simulink subsystem "TrajectoryLinkController"  (R2022b)
settings: Solver=VariableStepAuto  StartTime=0.0  StopTime=10.0  RelTol=1e-3
model mask{Tsampling=Tsampling, KpDiscrete=K(1,1), KdDiscrete=K(1,2), KiDiscrete=K(1,3), KpContinuous=K(1,1), KdContinuous=K(1,2), KiContinuous=K(1,3), ContinuousController=on}
  mask prompts: ContinuousController "Simulate Continuous Controller"
values from neighbouring files (symbols this model uses):
  Tsampling = 1e-3    (= 0.001)    [SimulationInput.m]    (also in SimulinkParameters.m; overleaf_sim.m; test_my_sim_class.m)
libraries: slpidlib x1
settings Model: Creator=papaveneti  LastModifiedBy=papaveneti

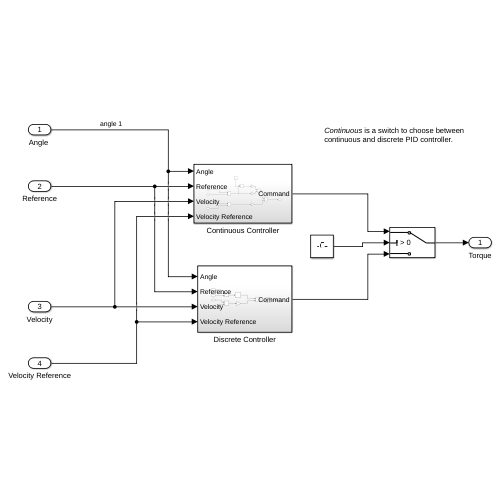
[thumbnail: Simulink's stored preview of the top-level diagram]
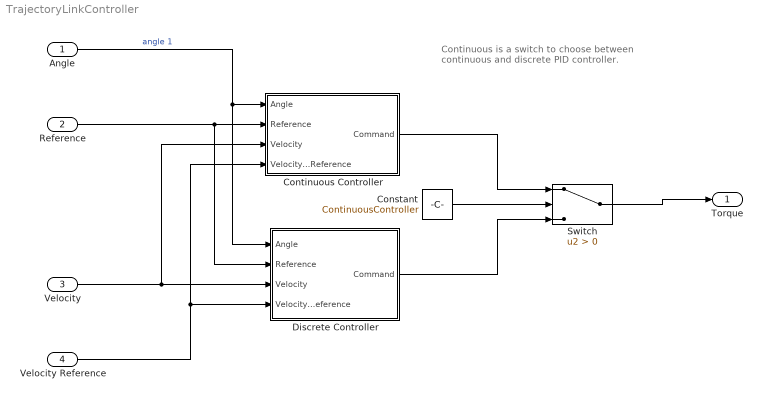
== system TrajectoryLinkController ==
  note: Continuous is a switch to choose between
      | continuous and discrete PID controller.
  "Angle " : Inport
  Reference : Inport  Port=2
  Velocity : Inport  Port=3
  Velocity Reference : Inport  Port=4
  Constant : Constant  Value=ContinuousController
  Continuous Controller : Subsystem
  Discrete Controller : Subsystem
  Switch : Switch  Criteria=u2 > Threshold  SaturateOnIntegerOverflow=off  InputSameDT=off
  Torque : Outport
  wires:
  Velocity Reference/1 -> Continuous Controller/4(Velocity Reference), Discrete Controller/4(Velocity Reference)
  Reference/1 -> Continuous Controller/2(Reference), Discrete Controller/2(Reference)
  Discrete Controller/1(Command) -> Switch/3
  Switch/1 -> Torque/1
  Continuous Controller/1(Command) -> Switch/1
  Velocity/1 -> Discrete Controller/3(Velocity), Continuous Controller/3(Velocity)
  "Angle "/1 -> Continuous Controller/1("Angle "), Discrete Controller/1(Angle)  "angle 1"
  Constant/1 -> Switch/2

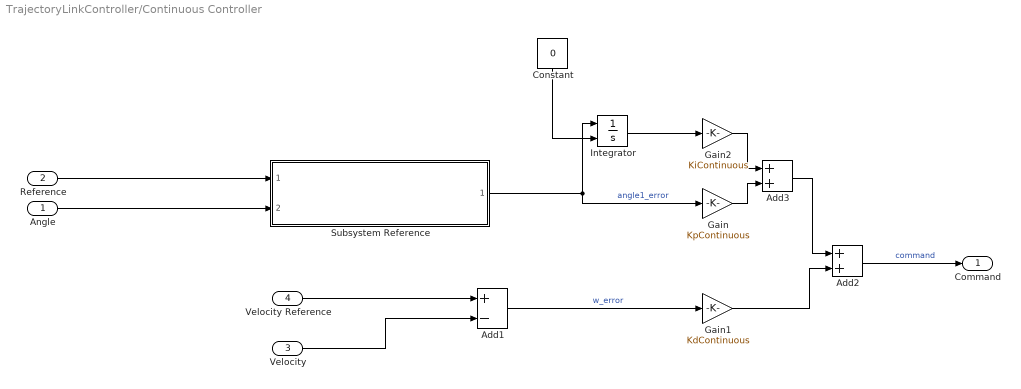
== system TrajectoryLinkController/Continuous Controller ==
  "Angle " : Inport
  Reference : Inport  Port=2
  Velocity : Inport  Port=3
  Velocity Reference : Inport  Port=4
  Add1 : Sum  Inputs=+-
  Add2 : Sum
  Add3 : Sum
  Constant : Constant  Value=0
  Gain : Gain  Gain=KpContinuous
  Gain1 : Gain  Gain=KdContinuous
  Gain2 : Gain  Gain=KiContinuous
  Integrator : Integrator  InitialConditionSource=external
  Subsystem Reference : Subsystem  ReferencedSubsystem=shortest_angle_diff
  Command : Outport
  wires:
  Constant/1 -> Integrator/2
  Add3/1 -> Add2/1
  Gain/1 -> Add3/2
  Gain2/1 -> Add3/1
  Integrator/1 -> Gain2/1
  Velocity Reference/1 -> Add1/1
  Velocity/1 -> Add1/2
  Subsystem Reference/1 -> Integrator/1, Gain/1  "angle1_error"
  "Angle "/1 -> Subsystem Reference/2
  Add2/1 -> Command/1  "command"
  Gain1/1 -> Add2/2
  Add1/1 -> Gain1/1  "w_error"
  Reference/1 -> Subsystem Reference/1

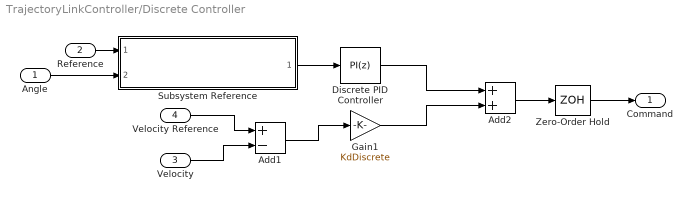
== system TrajectoryLinkController/Discrete Controller ==
  Angle : Inport
  Reference : Inport  Port=2
  Velocity : Inport  Port=3
  Velocity Reference : Inport  Port=4
  Add1 : Sum  Inputs=+-
  Add2 : Sum
  Discrete PID Controller : slpidlib/PID Controller  Controller=PI  Form=Parallel  TimeDomain=Discrete-time  UseExternalTs=off  SampleTime=Tsampling  IntegratorMethod=Forward Euler  FilterMethod=Forward Euler  ControllerParametersSource=internal  P=KpDiscrete  I=KiDiscrete  UseKiTs=off  D=0  N=100  UseFilter=off  TunerSelectOption=Transfer Function Based (PID Tuner App)  InitialConditionSource=internal  InitialConditionForIntegrator=0  InitialConditionForFilter=0  DifferentiatorICPrevScaledInput=0  ExternalReset=none  TrackingMode=off  Kt=1  LimitOutput=off  SatLimitsSource=internal  UpperSaturationLimit=inf  LowerSaturationLimit=-inf  LinearizeAsGain=off  AntiWindupMode=none  Kb=1  LimitIntegrator=off  UpperIntegratorSaturationLimit=inf  LowerIntegratorSaturationLimit=-inf  POutMin=[]  POutMax=[]  IOutMin=[]  IOutMax=[]  DOutMin=[]  DOutMax=[]  NOutMin=[]  NOutMax=[]  SumOutMin=[]  SumOutMax=[]  SaturationOutMin=[]  SaturationOutMax=[]  PParamMin=[]  PParamMax=[]  IParamMin=[]  IParamMax=[]  DParamMin=[]  DParamMax=[]  NParamMin=[]  NParamMax=[]  KbParamMin=[]  KbParamMax=[]  KtParamMin=[]  KtParamMax=[]  KbOutMin=[]  KbOutMax=[]  KtOutMin=[]  KtOutMax=[]  IntegratorOutMin=[]  IntegratorOutMax=[]  FilterOutMin=[]  FilterOutMax=[]  SumI1OutMin=[]  SumI1OutMax=[]  SumI2OutMin=[]  SumI2OutMax=[]  SumI3OutMin=[]  SumI3OutMax=[]  SumI4OutMin=[]  SumI4OutMax=[]  SumDOutMin=[]  SumDOutMax=[]  DifferentiatorOutMin=[]  DifferentiatorOutMax=[]  FilterDiffOutCoefMin=[]  FilterDiffOutCoefMax=[]  ReciprocalOutMin=[]  ReciprocalOutMax=[]  SumDenOutMin=[]  SumDenOutMax=[]  SumNumOutMin=[]  SumNumOutMax=[]  DivideOutMin=[]  DivideOutMax=[]  UdiffTsProdOutMin=[]  UdiffTsProdOutMax=[]  NTsProdOutMin=[]  NTsProdOutMax=[]  UintegralTsProdOutMin=[]  UintegralTsProdOutMax=[]  UngainTsProdOutMin=[]  UngainTsProdOutMax=[]  ClampingZeroOutDataTypeStr=Inherit: Inherit via back propagation  ClampingZeroOutMin=[]  ClampingZeroOutMax=[]  FilterDenConstantOutDataTypeStr=Inherit: Inherit via back propagation  FilterDenConstantOutMin=[]  FilterDenConstantOutMax=[]  PCopyOutDataTypeStr=Inherit: Inherit via back propagation  PCopyOutMin=[]  PCopyOutMax=[]  NCopyOutDataTypeStr=Inherit: Inherit via back propagation  NCopyOutMin=[]  NCopyOutMax=[]  IntegratorContinuousStateAttributes=''  IntegratorStateMustResolveToSignalObject=off  IntegratorRTWStateStorageClass=Auto  FilterContinuousStateAttributes=''  FilterStateMustResolveToSignalObject=off  FilterRTWStateStorageClass=Auto  ParallelPVariant=InternalParameters  IdealPVariant=Disabled  IVariant=InternalParameters  DVariant=Disabled  IntegratorVariant=Discrete  SatVariant=Disabled  AWVariant=Passthrough  PCopyVariant=Disabled  TRVariant=Disabled  FdbkBlocksVariant=Forward  IdealPFdbkVariant=Disabled  SatFdbkVariant=Disabled  DerivativeFilterVariant=Disabled  NVariant=Disabled  NCopyVariant=Disabled_SignalSpec  FilterICVariant=Disabled  IntegratorICVariant=InternalICs  ExternalResetVariant=Disabled  TRSumVariant=Passthrough  SumFdbkVariant=Disabled  SumVariant=Sum_PI  TsampFilterVariant=InternalTs  TsampNgainVariant=Passthrough  TsampIntegralVariant=Passthrough  ExternalSaturationOutDataTypeStr=Inherit: Same as second input
      settings: LibrarySourceBlock=simulink/Discrete/Discrete PID Controller
  Gain1 : Gain  Gain=KdDiscrete
  Subsystem Reference : Subsystem  ReferencedSubsystem=shortest_angle_diff
  Zero-Order Hold : ZeroOrderHold  SampleTime=Tsampling
  Command : Outport
  wires:
  Reference/1 -> Subsystem Reference/1
  Angle/1 -> Subsystem Reference/2
  Subsystem Reference/1 -> Discrete PID Controller/1
  Velocity Reference/1 -> Add1/1
  Velocity/1 -> Add1/2
  Add1/1 -> Gain1/1
  Gain1/1 -> Add2/2
  Discrete PID Controller/1 -> Add2/1
  Add2/1 -> Zero-Order Hold/1
  Zero-Order Hold/1 -> Command/1
